simulink model "GOPIO"  (R2024a)
settings: Solver=FixedStepAuto  StartTime=0.0  StopTime=inf  RelTol=1e-3  EnableMultiTasking=on
libraries: stm32f4xxblockslib x6, simulink x2, mcbcontrolslib x2, eeTransforms x1, simulink_extras x1, stm32blockslib x1
settings Model: Creator=wsl  LastModifiedBy=wsl
settings SolverCC: AutoInsertRateTranBlk=on
settings OptimizationCC: EnhancedBackFolding=on  PassReuseOutputArgsAs=Individual arguments  ZeroExternalMemoryAtStartup=off  ZeroInternalMemoryAtStartup=off  MaxStackSize=64  OptimizeBlockOrder=speed  DifferentSizesBufferReuse=on  OptimizationCustomize=off  EfficientTunableParamExpr=on
settings DebuggingCC: ParameterTunabilityLossMsg=error
settings HardwareCC: ProdBitPerPointer=32  ProdBitPerSizeT=32  ProdBitPerPtrDiffT=32  ProdLargestAtomicInteger=Long  ProdLargestAtomicFloat=Double  ProdWordSize=32  ProdLongLongMode=on  ProdHWDeviceType=ARM Compatible->ARM Cortex-M
settings SFSimCC: MATLABDynamicMemAlloc=off
settings RTWCC: Description=Embedded Coder  SystemTargetFile=ert.tlc  HardwareBoard=STM32F4xx Based  TemplateMakefile=ert_default_tmf  Toolchain=GNU Tools for ARM Embedded Processors
settings CodeAppCC: ForceParamTrailComments=on  IgnoreCustomStorageClasses=off  OperatorAnnotations=on  SimulinkDataObjDesc=on  SFDataObjDesc=on  InsertBlockDesc=on
settings ERTTargetCC: TargetLangStandard=C99 (ISO)  CodeReplacementLibrary=ARM Cortex-M  ExtModeTransport=3  ExtModeStaticAlloc=on  ExtModeStaticAllocSize=2048  ExtModeMexFile=ext_xcp  ExtModeIntrfLevel=Level2 - Open

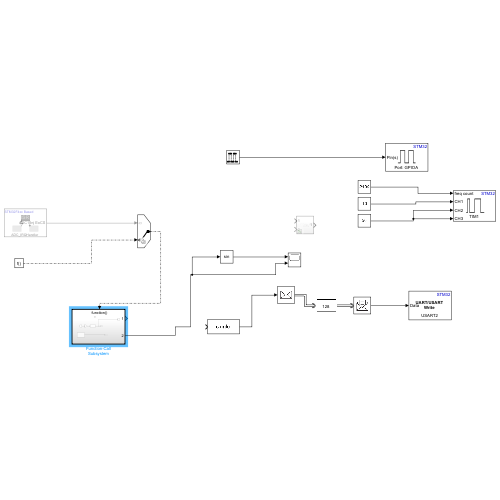
[thumbnail: Simulink's stored preview of the top-level diagram]
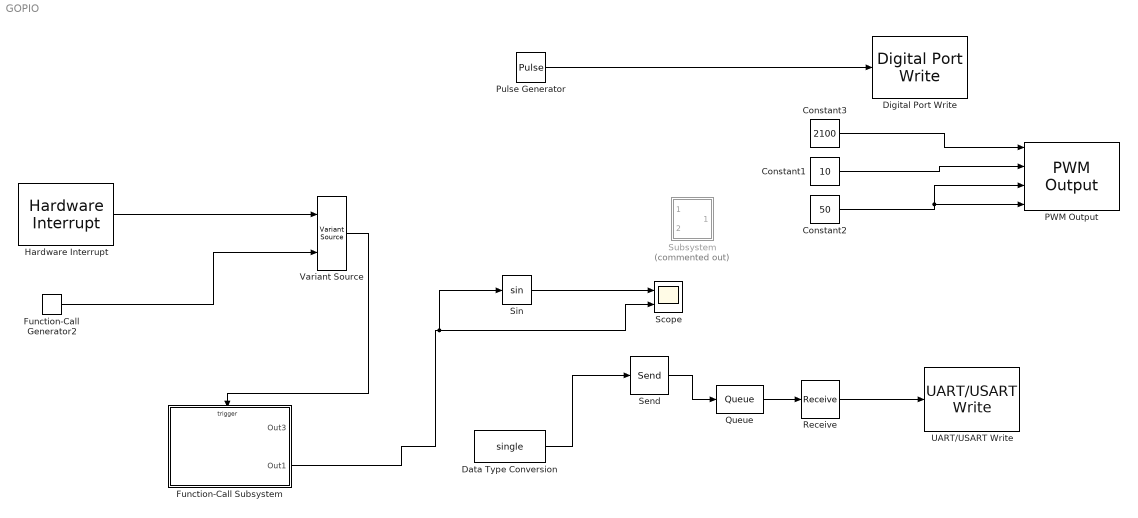
== system GOPIO ==
  Constant1 : Constant  Value=10
  Constant2 : Constant  Value=50
  Constant3 : Constant  Value=2100
  Data Type Conversion : DataTypeConversion  OutDataTypeStr=single  SaturateOnIntegerOverflow=off  RndMeth=Floor
  Digital Port Write : stm32f4xxblockslib/Digital Port Write  PortName=GPIOA  PinNumber=[5]  ReadOperation=off  IOAsArray=on  EnableSimPort=off
  Function-Call Generator2 : simulink/Ports & Subsystems/Function-Call Generator  sample_time=0.00005  numberOfIterations=1  DisallowWideOutput=off
  Function-Call Subsystem : Subsystem  TreatAsAtomicUnit=on
  Hardware Interrupt : stm32f4xxblockslib/Hardware Interrupt  ISRGroup=Analog to digital converter (ADC)  ISRName=ADC_IRQHandler  ISRNumber=33  EventsList={ 'off', 'ADC1 OVR', '1'; 'off', 'ADC1 Reg EoCS', '2'; 'on', 'ADC1 Inj EoCS', '3'; 'off', 'ADC1 Watchdog', '4'; 'off', 'ADC2 OVR', '5'; 'off', 'ADC2 Reg EoCS', '6'; 'off', 'ADC2 Inj EoCS', '7'; 'off', 'ADC2 Watchdog', '8'; 'off', 'ADC3 OVR', '9'; 'off', 'ADC3 Reg EoCS', '10'; 'off', 'ADC3 Inj EoCS', '11'; 'off', 'ADC3 Watchdog', '12'; 'off', 'Custom event', '13' }  SelectedEvents={'ADC1 Inj EoCS'}  TaskPriority=30  DisablePreemption=off  ClearInterruptFlagsAtEndOfEvent=off  InterruptDefinitionFile=$(TARGET_ROOT)/registry/interrupts/STM32F4xxBased_interrupts.xml  HardwareBoard=STM32F4xx Based  EnableSimPort=off
  PWM Output : stm32f4xxblockslib/PWM Output  TimerModule=TIM1  DutycycleUnits=Percentage  EnableChannel1=on  EnableChannel2=on  EnableChannel3=on  EnableChannel4=off  EnableCounterInput=off  EnableMainOutputInput=off  EnableFrequencyInput=on  SetRCAfterCE=on  OutputDirection=off  OutputMainOutputEnableStatus=off  SampleTime=0.1  EnableSimPort=off  EnableUpdateEvent=off  EnableCaptureCompare1Event=off  EnableCaptureCompare2Event=off  EnableCaptureCompare3Event=off  EnableCaptureCompare4Event=off  EnableTriggerEvent=off  EnableBreakEvent=off  ProcessorFamily=STM32F4  hoistedMaskSrc=ECSoC/ECSimCodegen/PWM Output
  Pulse Generator : DiscretePulseGenerator  Period=10  PulseWidth=5  SampleTime=0.1
  Queue : Queue  InputPortMessageModes=m  OutputPortMessageModes=m  OverwriteOldest=on  Capacity=128
  Receive : Receive  InputPortMessageModes=m  UseInternalQueue=off  QueueOverwriting=on  QueueLength=1  QueueType=LIFO
  Scope : Scope  NumInputPorts=2
  Send : Send  OutputPortMessageModes=m
  Sin : Trigonometry  ApproximationMethod=Lookup  TableDataTypeStr=fixdt(1,16,0)
  Subsystem : Subsystem  Commented=on
  UART/USART Write : stm32blockslib/UART//USART Write  UARTModule=USART2  LengthOfDataToSend=off  BlockingMode=off  BlockingTimeout=0.1  OutputStatus=off
      settings: LibrarySourceBlock=stm32f4xxblockslib/UART//USART Write
  Variant Source : VariantSource  VariantControlMode=sim codegen switching  OutputFunctionCall=on
  wires:
  Hardware Interrupt/1 -> Variant Source/1
  Variant Source/1 -> Function-Call Subsystem/Trigger
  Function-Call Generator2/1 -> Variant Source/2
  Constant3/1 -> PWM Output/1
  Constant2/1 -> PWM Output/3, PWM Output/4
  Constant1/1 -> PWM Output/2
  Pulse Generator/1 -> Digital Port Write/1
  Data Type Conversion/1 -> Send/1
  Function-Call Subsystem/2(Out1) -> Sin/1, Scope/2
  Queue/1 -> Receive/1
  Receive/1 -> UART/USART Write/1
  Send/1 -> Queue/1
  Sin/1 -> Scope/1

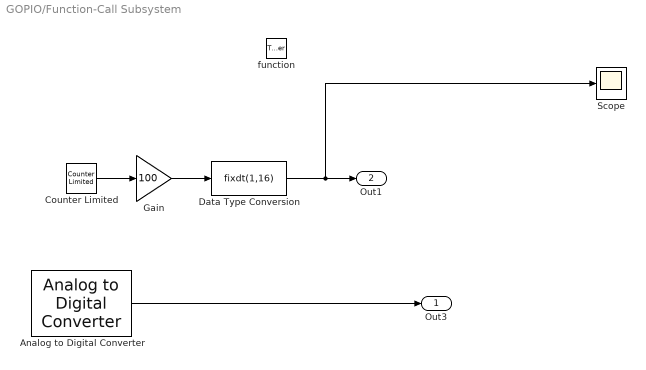
== system GOPIO/Function-Call Subsystem ==
  function : TriggerPort  TriggerType=function-call  VariantControl=(inherit)
  Analog to Digital Converter : stm32f4xxblockslib/Analog to Digital Converter  ADCModule=ADC1  ConversionGroup=Injected  TriggerMode=Read results only  NumberOfConversions=2  EnableBufferConv=off  BufferLength=1  OutputStatus=off  SampleTime=-1  EnableSimPort=off
  Counter Limited : simulink/Sources/Counter Limited  uplimit=20000000  tsamp=-1
  Data Type Conversion : DataTypeConversion  OutMin=[-pi]  OutMax=[pi]  OutDataTypeStr=fixdt(1,16)  SaturateOnIntegerOverflow=off  RndMeth=Floor
  Gain : Gain  Gain=100
  Scope : Scope
  Out3 : Outport
  Out1 : Outport  Port=2
  wires:
  Analog to Digital Converter/1 -> Out3/1
  Counter Limited/1 -> Gain/1
  Data Type Conversion/1 -> Scope/1, Out1/1
  Gain/1 -> Data Type Conversion/1

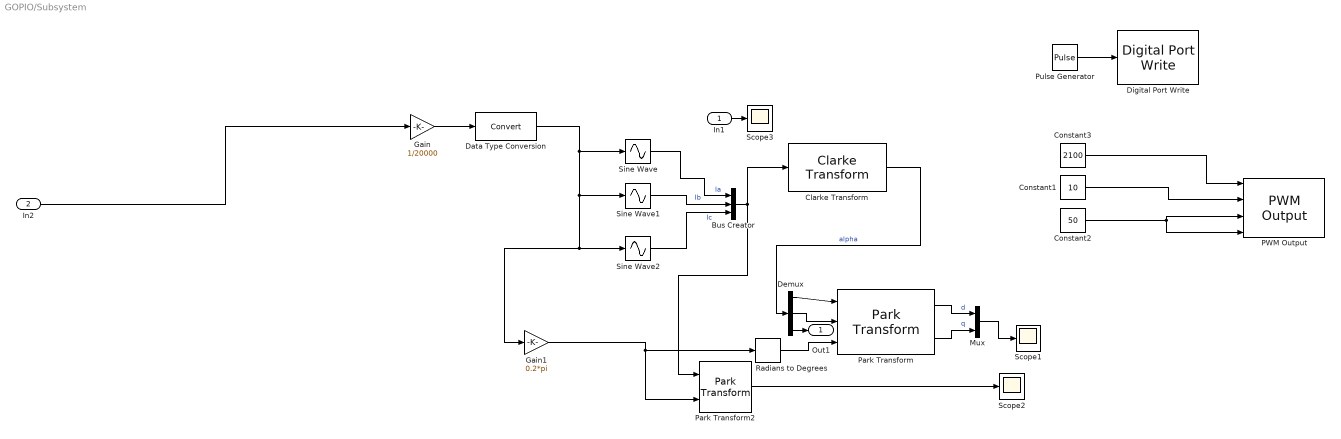
== system GOPIO/Subsystem ==
  In1 : Inport
  In2 : Inport  Port=2
  Bus Creator : BusCreator  Inputs=3
  Clarke Transform : mcbcontrolslib/Clarke Transform  VariantControl=Variant2  PhaseInput=Three inputs  EnPowerInv=off
      settings: LibrarySourceBlock=mcbhdllib/Controls/Math Transforms/Clarke Transform
  Constant1 : Constant  Value=10
  Constant2 : Constant  Value=50
  Constant3 : Constant  Value=2100
  Data Type Conversion : DataTypeConversion  SaturateOnIntegerOverflow=off  RndMeth=Floor
  Demux : Demux  Outputs=3
  Digital Port Write : stm32f4xxblockslib/Digital Port Write  PortName=GPIOA  PinNumber=[5]  ReadOperation=off  IOAsArray=on  EnableSimPort=off
  Gain : Gain  Gain=1/20000
  Gain1 : Gain  Gain=0.2*pi
  Mux : Mux  Inputs=2
  PWM Output : stm32f4xxblockslib/PWM Output  TimerModule=TIM1  DutycycleUnits=Percentage  EnableChannel1=on  EnableChannel2=on  EnableChannel3=on  EnableChannel4=off  EnableCounterInput=off  EnableMainOutputInput=off  EnableFrequencyInput=on  SetRCAfterCE=on  OutputDirection=off  OutputMainOutputEnableStatus=off  SampleTime=0.1  EnableSimPort=off  EnableUpdateEvent=off  EnableCaptureCompare1Event=off  EnableCaptureCompare2Event=off  EnableCaptureCompare3Event=off  EnableCaptureCompare4Event=off  EnableTriggerEvent=off  EnableBreakEvent=off  ProcessorFamily=STM32F4  hoistedMaskSrc=ECSoC/ECSimCodegen/PWM Output
  Park Transform : mcbcontrolslib/Park Transform  PhaseInput=Two inputs  AxisAlignment=Q-axis  ThetaInput=Electrical position  AngleInput=Degrees  N_points=1024
      settings: LibrarySourceBlock=mcbhdllib/Controls/Math Transforms/Park Transform
  Park Transform2 : eeTransforms/Park Transform  AxisAlignment=Q-axis  PowerInvariant=off
      settings: LibrarySourceBlock=|
      | ee_sl_lib/Mathematical
      | Transforms/Park Transform
  Pulse Generator : DiscretePulseGenerator  Period=10  PulseWidth=5  SampleTime=0.1
  Radians to Degrees : simulink_extras/Transformations/Radians to Degrees
  Scope1 : Scope
  Scope2 : Scope
  Scope3 : Scope
  Sine Wave : Sin  TimeSource=Use external signal  Amplitude=10  Frequency=0.2*pi  Phase=pi/2  SampleTime=0
  Sine Wave1 : Sin  TimeSource=Use external signal  Amplitude=10  Frequency=0.2*pi  Phase=-2/3*pi+pi/2  SampleTime=0
  Sine Wave2 : Sin  TimeSource=Use external signal  Amplitude=10  Frequency=0.2*pi  Phase=2/3*pi+pi/2  SampleTime=0
  Out1 : Outport
  wires:
  Demux/2 -> Park Transform/2
  Sine Wave2/1 -> Bus Creator/3  "Ic"
  Pulse Generator/1 -> Digital Port Write/1
  Demux/1 -> Park Transform/1
  Park Transform/2 -> Mux/2  "q"
  Park Transform2/1 -> Scope2/1
  Constant2/1 -> PWM Output/3, PWM Output/4
  Gain/1 -> Data Type Conversion/1
  Constant1/1 -> PWM Output/2
  Clarke Transform/1 -> Demux/1  "alpha"
  Sine Wave1/1 -> Bus Creator/2  "Ib"
  Bus Creator/1 -> Park Transform2/1, Clarke Transform/1
  Demux/3 -> Out1/1
  Constant3/1 -> PWM Output/1
  Data Type Conversion/1 -> Gain1/1, Sine Wave2/1, Sine Wave1/1, Sine Wave/1
  Mux/1 -> Scope1/1
  Radians to Degrees/1 -> Park Transform/3
  Park Transform/1 -> Mux/1  "d"
  Gain1/1 -> Park Transform2/2, Radians to Degrees/1
  Sine Wave/1 -> Bus Creator/1  "Ia"
  In1/1 -> Scope3/1
  In2/1 -> Gain/1
